simulink model "Bands4"  (R2018a)
settings: Solver=VariableStepAuto  StartTime=0.0  StopTime=0.001  RelTol=1e-3
undefined symbols (not defined in the file): fdesignblkfcn, G1, G2, G3, G4, gcbh, get, T
libraries: dspsrcs4 x1, dspxfrm3 x1, dspobslib x1
settings Model: Creator=Daniel  LastModifiedBy=Daniel

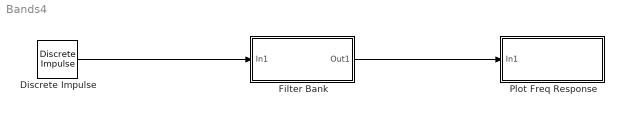
== system Bands4 ==
  Discrete Impulse : dspsrcs4/Discrete  Impulse  Delay=0  SampleTime=T  FrameSample=128  OutputFrames=off  dataType=double  isSigned=on  wordLen=16  udDataType=sfix(16)  fracBitsMode=Best precision  numFracBits=15  OutDataTypeStr=double  LastOutDataTypeStr=double
  "Filter Bank " : Subsystem
  Plot Freq Response : Subsystem
  wires:
  Discrete Impulse/1 -> "Filter Bank "/1(In1)
  "Filter Bank "/1(Out1) -> Plot Freq Response/1(In1)

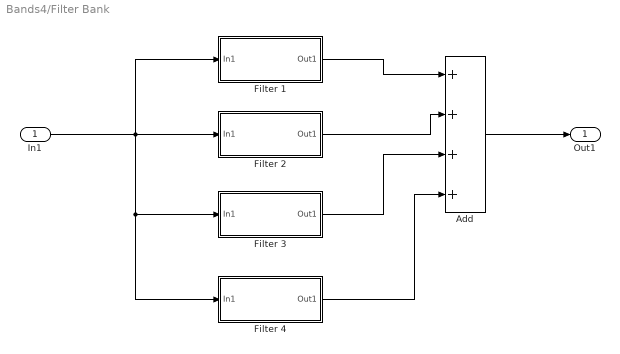
== system Bands4/Filter Bank  ==
  In1 : Inport
  Add : Sum  Inputs=++++
  Filter 1 : Subsystem
  Filter 2 : Subsystem
  Filter 3 : Subsystem
  Filter 4 : Subsystem
  Out1 : Outport
  wires:
  In1/1 -> Filter 3/1(In1), Filter 4/1(In1), Filter 1/1(In1), Filter 2/1(In1)
  Add/1 -> Out1/1
  Filter 1/1(Out1) -> Add/1
  Filter 2/1(Out1) -> Add/2
  Filter 3/1(Out1) -> Add/3
  Filter 4/1(Out1) -> Add/4

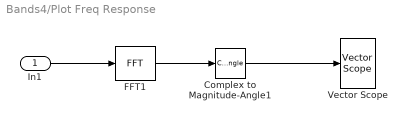
== system Bands4/Plot Freq Response ==
  In1 : Inport
  Complex to Magnitude-Angle1 : ComplexToMagnitudeAngle  Output=Magnitude
  FFT1 : dspxfrm3/FFT  FFTImplementation=Auto  CompMethod=Table lookup  TableOpt=NEW  TableOptActive=Speed  BitRevOrder=off  Normalize=off  InheritFFTLength=on  FFTLength=64  WrapInput=on  roundingMode=Floor  overflowMode=off  firstCoeffDataTypeStr=Inherit: Same word length as input  firstCoeffLastDataTypeStr=Inherit: Same word length as input  outputMin=[]  outputMax=[]
  Vector Scope : dspobslib/Vector Scope  ScopeProperties=off  Domain=Frequency  HorizSpan=1  DisplayProperties=off  AxisGrid=on  Memory=off  FrameNumber=off  AxisLegend=off  AxisZoom=off  OpenScopeAtSimStart=on  OpenScopeImmediately=off  FigPos=get(0,'defaultfigureposition')  AxisProperties=on  XUnits=Hertz  XRange=[0...Fs/2]  InheritXIncr=on  XIncr=1  XLabel=Samples  XLimit=Auto  XMin=0  XMax=1  XStart=0  YUnits=dB  YLabel=|Magnitude (dB)|  LineProperties=off  XAxisParamsVer=6.9
      settings: SourceProductName=DSP System Toolbox  SourceProductBaseCode=DS  YMin=0.0723692553519949  YMax=69.3188381671759
  wires:
  In1/1 -> FFT1/1
  FFT1/1 -> Complex to Magnitude-Angle1/1
  Complex to Magnitude-Angle1/1 -> Vector Scope/1

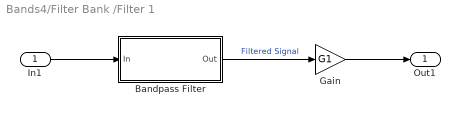
== system Bands4/Filter Bank /Filter 1 ==
  In1 : Inport
  Bandpass Filter : Subsystem  DialogController=fdesignblkfcn  InitFcn=fdesignblkfcn(gcbh, {'InitFcn'});  mask(Bandpass Filter){}
      mask help: Design a bandpass filter
      settings: CopyFcn=fdesignblkfcn(gcbh, {'CopyFcn'});
      mask Help: helpview(mapfilelocation('dsp'), 'dspbandpassfilter');
      mask Display: disp('Bandpass');
  Gain : Gain  Gain=G1
  Out1 : Outport
  wires:
  Bandpass Filter/1(Out) -> Gain/1  "Filtered Signal"
  In1/1 -> Bandpass Filter/1(In)
  Gain/1 -> Out1/1

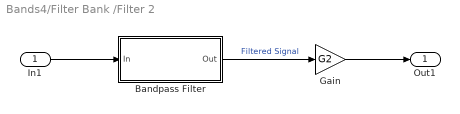
== system Bands4/Filter Bank /Filter 2 ==
  In1 : Inport
  Bandpass Filter : Subsystem  DialogController=fdesignblkfcn  InitFcn=fdesignblkfcn(gcbh, {'InitFcn'});  mask(Bandpass Filter){}
      mask help: Design a bandpass filter
      settings: CopyFcn=fdesignblkfcn(gcbh, {'CopyFcn'});
      mask Help: helpview(mapfilelocation('dsp'), 'dspbandpassfilter');
      mask Display: disp('Bandpass');
  Gain : Gain  Gain=G2
  Out1 : Outport
  wires:
  Bandpass Filter/1(Out) -> Gain/1  "Filtered Signal"
  In1/1 -> Bandpass Filter/1(In)
  Gain/1 -> Out1/1

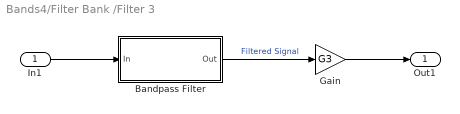
== system Bands4/Filter Bank /Filter 3 ==
  In1 : Inport
  Bandpass Filter : Subsystem  DialogController=fdesignblkfcn  InitFcn=fdesignblkfcn(gcbh, {'InitFcn'});  mask(Bandpass Filter){}
      mask help: Design a bandpass filter
      settings: CopyFcn=fdesignblkfcn(gcbh, {'CopyFcn'});
      mask Help: helpview(mapfilelocation('dsp'), 'dspbandpassfilter');
      mask Display: disp('Bandpass');
  Gain : Gain  Gain=G3
  Out1 : Outport
  wires:
  Bandpass Filter/1(Out) -> Gain/1  "Filtered Signal"
  In1/1 -> Bandpass Filter/1(In)
  Gain/1 -> Out1/1

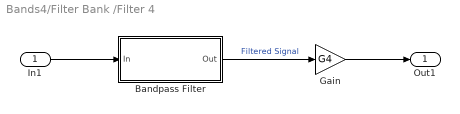
== system Bands4/Filter Bank /Filter 4 ==
  In1 : Inport
  Bandpass Filter : Subsystem  DialogController=fdesignblkfcn  InitFcn=fdesignblkfcn(gcbh, {'InitFcn'});  mask(Bandpass Filter){}
      mask help: Design a bandpass filter
      settings: CopyFcn=fdesignblkfcn(gcbh, {'CopyFcn'});
      mask Help: helpview(mapfilelocation('dsp'), 'dspbandpassfilter');
      mask Display: disp('Bandpass');
  Gain : Gain  Gain=G4
  Out1 : Outport
  wires:
  Bandpass Filter/1(Out) -> Gain/1  "Filtered Signal"
  In1/1 -> Bandpass Filter/1(In)
  Gain/1 -> Out1/1

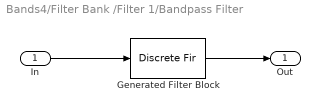
== system Bands4/Filter Bank /Filter 1/Bandpass Filter ==
  In : Inport
  Generated Filter Block : DiscreteFir  Tag=BlockMethodSubSystem  Coefficients=[0.00133278612923119419 -0.00331875460655659546 -0.0043565325545410127 -0.00582980177046569289 -0.00677257689549515263 -0.00666038821048054071 -0.00534876114611354189 -0.00309498598435489596 -0.000497218550964517508 0.00168911426787105392 0.00280790262215445006 0.00254254945855138595 0.00105026625064580837 -0.00107739201307651832 -0.00301923291404763549 -0.00403179806731172354 -0.00373960093990319221 -0.00229452322320222463 -0.000329736993283772956 0.00128092784894239344 0.0017743067668979243 0.000817354200727052446 -0.00133252940358492703 -0.00390651271618730651 -0.00591771943696455319 -0.00656487236307345089 -0.00557954869720924968 -0.00337296462099866004 -0.000901634255472844601 0.000702545970788563852 0.00060403734184114185 -0.00136601697689596869 -0.00459356006885095532 -0.00789298102307913613 -0.00996925578026862727 -0.00996052718167413434 -0.00783258809293354598 -0.00445495814879968283 -0.00128579092314304723 0.000198561551184634486 -0.000857508925310963908 -0.00430181480018963953 -0.00895317091429130227 -0.0130144425963712972 -0.0148289388868921099 -0.0135507838862912438 -0.00959759454149750231 -0.0045524336413870865 -0.000590480980185252189 0.000402957134257909868 -0.00234686865001167057 -0.00807970353376383579 -0.0146980473221125472 -0.0195398271092478773 -0.0204634680894347463 -0.0168000985733509217 -0.00977609816099122945 -0.00216856626599984566 0.00271998399806409451 0.00241176995964558546 -0.00361282367739521265 -0.013483161295937721 -0.023465611895269245 -0.0293226200086963533 -0.0280408846926225065 -0.0192519853544229035 -0.00573934499296634322 0.00728612140105600482 0.0139924146345874068 0.0102373212639982648 -0.00445875990747033723 -0.0260669794386082301 -0.0467877021886915698 -0.0572697043412922768 -0.0496733388904965212 -0.0205709642359263555 0.0273342803691389649 0.0853418117581927482 0.140837578627084653 0.180737432426107847 0.195243690370153017 0.180737432426107847 0.140837578627084653 0.0853418117581927482 0.0273342803691389649 -0.0205709642359263555 -0.0496733388904965212 -0.0572697043412922768 -0.0467877021886915698 -0.0260669794386082301 -0.00445875990747033723 0.0102373212639982648 0.0139924146345874068 0.00728612140105600482 -0.00573934499296634322 -0.0192519853544229035 -0.0280408846926225065 -0.0293226200086963533 -0.023465611895269245 -0.013483161295937721 -0.00361282367739521265 0.00241176995964558546 0.00271998399806409451 -0.00216856626599984566 -0.00977609816099122945 -0.0168000985733509217 -0.0204634680894347463 -0.0195398271092478773 -0.0146980473221125472 -0.00807970353376383579 -0.00234686865001167057 0.000402957134257909868 -0.000590480980185252189 -0.0045524336413870865 -0.00959759454149750231 -0.0135507838862912438 -0.0148289388868921099 -0.0130144425963712972 -0.00895317091429130227 -0.00430181480018963953 -0.000857508925310963908 0.000198561551184634486 -0.00128579092314304723 -0.00445495814879968283 -0.00783258809293354598 -0.00996052718167413434 -0.00996925578026862727 -0.00789298102307913613 -0.00459356006885095532 -0.00136601697689596869 0.00060403734184114185 0.000702545970788563852 -0.000901634255472844601 -0.00337296462099866004 -0.00557954869720924968 -0.00656487236307345089 -0.00591771943696455319 -0.00390651271618730651 -0.00133252940358492703 0.000817354200727052446 0.0017743067668979243 0.00128092784894239344 -0.000329736993283772956 -0.00229452322320222463 -0.00373960093990319221 -0.00403179806731172354 -0.00301923291404763549 -0.00107739201307651832 0.00105026625064580837 0.00254254945855138595 0.00280790262215445006 0.00168911426787105392 -0.000497218550964517508 -0.00309498598435489596 -0.00534876114611354189 -0.00666038821048054071 -0.00677257689549515263 -0.00582980177046569289 -0.0043565325545410127 -0.00331875460655659546 0.00133278612923119419]  InputProcessing=Columns as channels (frame based)
  Out : Outport
  wires:
  In/1 -> Generated Filter Block/1
  Generated Filter Block/1 -> Out/1

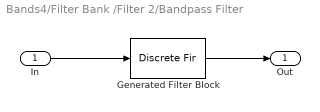
== system Bands4/Filter Bank /Filter 2/Bandpass Filter ==
  In : Inport
  Generated Filter Block : DiscreteFir  Tag=BlockMethodSubSystem  Coefficients=[-0.0029966902436686961 0.000163740294120938976 0.00193397286969325291 0.00242655640813694597 0.00110697236682085571 2.45270978643425359e-05 0.000899541149797445077 0.00210317797713385898 0.00036449241930275962 -0.00420136726437577053 -0.00666047844818571256 -0.00268846119189026546 0.0052493595663690067 0.0094468000566339666 0.00552303092229697139 -0.00230720482468481976 -0.00618214514497822387 -0.00378003347202423559 -0.000138930764970942981 -0.000172159388794992528 -0.00220414507068683249 -0.00117797815010535424 0.00337048484005184968 0.00611399039405029383 0.00335929020271850953 -0.00156850765949116179 -0.00289249528651256424 -0.000526689638721184014 4.75086518841008376e-05 -0.00360903210425100656 -0.00641950237536057303 -0.00259328301058467251 0.00539858357060056006 0.00894830687543468617 0.00449727054309354956 -0.00168450172391017392 -0.00227126137633249306 0.000900954453604899011 -1.61433361490476954e-05 -0.00648876846275591845 -0.0100280345509410514 -0.00367974053739447606 0.00719335200065133844 0.0108889208018009189 0.00479809191003415392 -0.0013669645679542492 0.000292745088516118443 0.00428032622294609311 -1.57622073685547101e-05 -0.011297844231085815 -0.015691845785276725 -0.00531465178055592295 0.00951143761033315487 0.0129165273155258161 0.00461590802329728354 -0.000468890249699975776 0.00540361975229013483 0.0103606487050574934 -2.60295909985121165e-05 -0.0191721922207331655 -0.0245912075022944182 -0.00774328217527216981 0.0125851329891607348 0.0145442779496458268 0.00302765214013625767 0.00185412088892863568 0.0169659674394883782 0.0235177324414267246 -4.01391400627775684e-05 -0.0359045831154521031 -0.0435271431704272183 -0.012868264309105891 0.0186739167089275994 0.0156202846971824835 -0.0036237790251913162 0.0101276225605185163 0.0596503519443067065 0.0763659759040795222 -4.26076983414284065e-05 -0.125606425964924689 -0.171541832483379619 -0.0616834888278260385 0.124533073844955905 0.215994825554424674 0.124533073844955905 -0.0616834888278260385 -0.171541832483379619 -0.125606425964924689 -4.26076983414284065e-05 0.0763659759040795222 0.0596503519443067065 0.0101276225605185163 -0.0036237790251913162 0.0156202846971824835 0.0186739167089275994 -0.012868264309105891 -0.0435271431704272183 -0.0359045831154521031 -4.01391400627775684e-05 0.0235177324414267246 0.0169659674394883782 0.00185412088892863568 0.00302765214013625767 0.0145442779496458268 0.0125851329891607348 -0.00774328217527216981 -0.0245912075022944182 -0.0191721922207331655 -2.60295909985121165e-05 0.0103606487050574934 0.00540361975229013483 -0.000468890249699975776 0.00461590802329728354 0.0129165273155258161 0.00951143761033315487 -0.00531465178055592295 -0.015691845785276725 -0.011297844231085815 -1.57622073685547101e-05 0.00428032622294609311 0.000292745088516118443 -0.0013669645679542492 0.00479809191003415392 0.0108889208018009189 0.00719335200065133844 -0.00367974053739447606 -0.0100280345509410514 -0.00648876846275591845 -1.61433361490476954e-05 0.000900954453604899011 -0.00227126137633249306 -0.00168450172391017392 0.00449727054309354956 0.00894830687543468617 0.00539858357060056006 -0.00259328301058467251 -0.00641950237536057303 -0.00360903210425100656 4.75086518841008376e-05 -0.000526689638721184014 -0.00289249528651256424 -0.00156850765949116179 0.00335929020271850953 0.00611399039405029383 0.00337048484005184968 -0.00117797815010535424 -0.00220414507068683249 -0.000172159388794992528 -0.000138930764970942981 -0.00378003347202423559 -0.00618214514497822387 -0.00230720482468481976 0.00552303092229697139 0.0094468000566339666 0.0052493595663690067 -0.00268846119189026546 -0.00666047844818571256 -0.00420136726437577053 0.00036449241930275962 0.00210317797713385898 0.000899541149797445077 2.45270978643425359e-05 0.00110697236682085571 0.00242655640813694597 0.00193397286969325291 0.000163740294120938976 -0.0029966902436686961]  InputProcessing=Columns as channels (frame based)
  Out : Outport
  wires:
  In/1 -> Generated Filter Block/1
  Generated Filter Block/1 -> Out/1

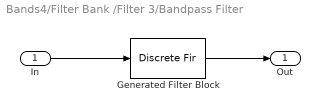
== system Bands4/Filter Bank /Filter 3/Bandpass Filter ==
  In : Inport
  Generated Filter Block : DiscreteFir  Tag=BlockMethodSubSystem  Coefficients=[0.00196163489536466725 -0.00298628646788819552 -0.00278841433951132305 0.00118017851193852807 0.00174129623447588601 -0.000764140617058064759 -0.000811796866947125679 -0.00115830628446497242 -0.00125492877726778203 0.00353006711623102872 0.0035663126623454648 -0.00579612858589233313 -0.00536820462098256627 0.00705019896726515483 0.00584297768150565319 -0.00666942986297104461 -0.00459599205616372918 0.00457094221052579703 0.00187918120458679776 -0.00136432475894594308 0.00139228697698347888 -0.00179958254997254589 -0.00394900501423298828 0.00365927196554522664 0.00467449566062221739 -0.00337745085864509876 -0.00313377021337711776 0.000976803130033732092 -0.00015186384583149937 0.0025647894492198493 0.00380763984243921629 -0.00563644287704273116 -0.00613358604146005577 0.00666088459373619102 0.00583928940557217578 -0.00482699386166717676 -0.00270421914616655098 0.000571695130607383518 -0.0021814649538956371 0.00446173934283700634 0.00674869948195539523 -0.0080221987856019944 -0.0087859130771532068 0.00822378357581123043 0.00695210212577722798 -0.00448586739824804927 -0.00153670404474663506 -0.00200439221980046756 -0.00543804827303336156 0.00858441466739485841 0.010904616367960876 -0.0121289430697496155 -0.0120154369368301178 0.0104371876372589354 0.00750421521135567673 -0.0034075130188455224 0.00146396326309186468 -0.00657038990086519347 -0.0114219364014046185 0.0152844182298202281 0.0177922448595748406 -0.0182985691894405229 -0.0167665403082698436 0.0129342108651963883 0.00718338903186476786 0.000179023296547248072 0.00841711787623867017 -0.0166914674573216439 -0.0241129906694968303 0.0295818667604102574 0.0323421910671751744 -0.0314432157059355497 -0.0265474045869606157 0.0172605456756602764 0.00382034846562357127 0.0133770746055091837 0.0335190098967853706 -0.0554665772344861349 -0.0780342247712595138 0.0996647713261604035 0.119125015589209376 -0.134943459219041273 -0.146195817993647698 0.15199264081956132 0.15199264081956132 -0.146195817993647698 -0.134943459219041273 0.119125015589209376 0.0996647713261604035 -0.0780342247712595138 -0.0554665772344861349 0.0335190098967853706 0.0133770746055091837 0.00382034846562357127 0.0172605456756602764 -0.0265474045869606157 -0.0314432157059355497 0.0323421910671751744 0.0295818667604102574 -0.0241129906694968303 -0.0166914674573216439 0.00841711787623867017 0.000179023296547248072 0.00718338903186476786 0.0129342108651963883 -0.0167665403082698436 -0.0182985691894405229 0.0177922448595748406 0.0152844182298202281 -0.0114219364014046185 -0.00657038990086519347 0.00146396326309186468 -0.0034075130188455224 0.00750421521135567673 0.0104371876372589354 -0.0120154369368301178 -0.0121289430697496155 0.010904616367960876 0.00858441466739485841 -0.00543804827303336156 -0.00200439221980046756 -0.00153670404474663506 -0.00448586739824804927 0.00695210212577722798 0.00822378357581123043 -0.0087859130771532068 -0.0080221987856019944 0.00674869948195539523 0.00446173934283700634 -0.0021814649538956371 0.000571695130607383518 -0.00270421914616655098 -0.00482699386166717676 0.00583928940557217578 0.00666088459373619102 -0.00613358604146005577 -0.00563644287704273116 0.00380763984243921629 0.0025647894492198493 -0.00015186384583149937 0.000976803130033732092 -0.00313377021337711776 -0.00337745085864509876 0.00467449566062221739 0.00365927196554522664 -0.00394900501423298828 -0.00179958254997254589 0.00139228697698347888 -0.00136432475894594308 0.00187918120458679776 0.00457094221052579703 -0.00459599205616372918 -0.00666942986297104461 0.00584297768150565319 0.00705019896726515483 -0.00536820462098256627 -0.00579612858589233313 0.0035663126623454648 0.00353006711623102872 -0.00125492877726778203 -0.00115830628446497242 -0.000811796866947125679 -0.000764140617058064759 0.00174129623447588601 0.00118017851193852807 -0.00278841433951132305 -0.00298628646788819552 0.00196163489536466725]  InputProcessing=Columns as channels (frame based)
  Out : Outport
  wires:
  In/1 -> Generated Filter Block/1
  Generated Filter Block/1 -> Out/1

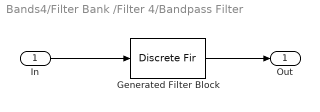
== system Bands4/Filter Bank /Filter 4/Bandpass Filter ==
  In : Inport
  Generated Filter Block : DiscreteFir  Tag=BlockMethodSubSystem  Coefficients=[-0.00294013978430311988 0.0114290942736278937 -0.0125637612669188773 0.0093715194565400263 -0.000963837498904158269 -0.00459544399890903562 0.00389934734173801381 5.36673366236276674e-05 -0.00129930697958306317 -0.00130625579592801998 0.00316252299269712336 -0.000537252522496357268 -0.00403796605824010679 0.00502271776211917365 -0.00134705986751200327 -0.00220721280025314246 0.00168542348779582882 0.000655745167688686075 5.99207162747558998e-05 -0.00381232984041724723 0.00516480725736678369 -0.000923329775585184044 -0.00477426506658664308 0.00559679932617655144 -0.00155666504557058576 -0.00118530635344824215 -0.000723972887676736397 0.00288658938890202664 0.000292894235418140851 -0.00665394086865600358 0.0082027821316034543 -0.00204289923283256219 -0.00502973958290784187 0.00541835882161673024 -0.0010079612103138149 2.62122979274945092e-05 -0.00455367933687486452 0.00676461027294797141 -0.000170980648444613427 -0.00975471419639770132 0.0116017454397041725 -0.00337266876285630037 -0.00448274816433389539 0.003461349466024226 0.00119000930078477134 0.00136129918821703967 -0.0104239329371323079 0.0128870895309000488 -0.00152161029658084198 -0.0130120979292555426 0.0149286204048315486 -0.00442428891823994693 -0.00283478812761097515 -0.00165813210803645444 0.00652374057130226601 0.00262959319275206773 -0.0196498758850854188 0.0227740164799063137 -0.00422864067116998296 -0.0166200414626759309 0.0177230034614148865 -0.00423343564928185812 0.000644188960532906868 -0.0137507319437919981 0.0194101252563012583 0.00362597655472521926 -0.0377473689135182158 0.0429970764101891972 -0.0101264180944409341 -0.0227096967499407013 0.0195723050026766279 0.00113044395635356195 0.0102934650615658339 -0.0574330503751945901 0.0725339695879020918 0.00417885940916125614 -0.128646777079804681 0.172446028249970157 -0.0601313480061003158 -0.128026633077345409 0.220219792616067278 -0.128026633077345409 -0.0601313480061003158 0.172446028249970157 -0.128646777079804681 0.00417885940916125614 0.0725339695879020918 -0.0574330503751945901 0.0102934650615658339 0.00113044395635356195 0.0195723050026766279 -0.0227096967499407013 -0.0101264180944409341 0.0429970764101891972 -0.0377473689135182158 0.00362597655472521926 0.0194101252563012583 -0.0137507319437919981 0.000644188960532906868 -0.00423343564928185812 0.0177230034614148865 -0.0166200414626759309 -0.00422864067116998296 0.0227740164799063137 -0.0196498758850854188 0.00262959319275206773 0.00652374057130226601 -0.00165813210803645444 -0.00283478812761097515 -0.00442428891823994693 0.0149286204048315486 -0.0130120979292555426 -0.00152161029658084198 0.0128870895309000488 -0.0104239329371323079 0.00136129918821703967 0.00119000930078477134 0.003461349466024226 -0.00448274816433389539 -0.00337266876285630037 0.0116017454397041725 -0.00975471419639770132 -0.000170980648444613427 0.00676461027294797141 -0.00455367933687486452 2.62122979274945092e-05 -0.0010079612103138149 0.00541835882161673024 -0.00502973958290784187 -0.00204289923283256219 0.0082027821316034543 -0.00665394086865600358 0.000292894235418140851 0.00288658938890202664 -0.000723972887676736397 -0.00118530635344824215 -0.00155666504557058576 0.00559679932617655144 -0.00477426506658664308 -0.000923329775585184044 0.00516480725736678369 -0.00381232984041724723 5.99207162747558998e-05 0.000655745167688686075 0.00168542348779582882 -0.00220721280025314246 -0.00134705986751200327 0.00502271776211917365 -0.00403796605824010679 -0.000537252522496357268 0.00316252299269712336 -0.00130625579592801998 -0.00129930697958306317 5.36673366236276674e-05 0.00389934734173801381 -0.00459544399890903562 -0.000963837498904158269 0.0093715194565400263 -0.0125637612669188773 0.0114290942736278937 -0.00294013978430311988]  InputProcessing=Columns as channels (frame based)
  Out : Outport
  wires:
  In/1 -> Generated Filter Block/1
  Generated Filter Block/1 -> Out/1
